simulink model "test_darko"  (R2021b)
settings: Solver=VariableStepAuto  StartTime=0.0  StopTime=100  RelTol=1e-3
values from neighbouring files (symbols this model uses):
  initial_state = [p_initial; v_initial; q_initial; omega_initial]    [systune_gain_scheduling.m]    (also in systune_variable_gain_scheduling_LPV.m)
  u_eq = [ua;ua;ub;ub]    [systune_gain_scheduling.m]    (also in systune_variable_gain_scheduling_LPV.m)
  w = [0;0;0]    [systune_gain_scheduling.m]    (also in systune_variable_gain_scheduling_LPV.m = [-i;0;0])
libraries: simulink_extras x5, aerolibanim x1, sharedtransform x1
settings Model: Creator=florian  LastModifiedBy=florian
settings SolverCC: AlgebraicLoopSolver=TrustRegion
settings DebuggingCC: SFMachineParentedDataDiag=warning

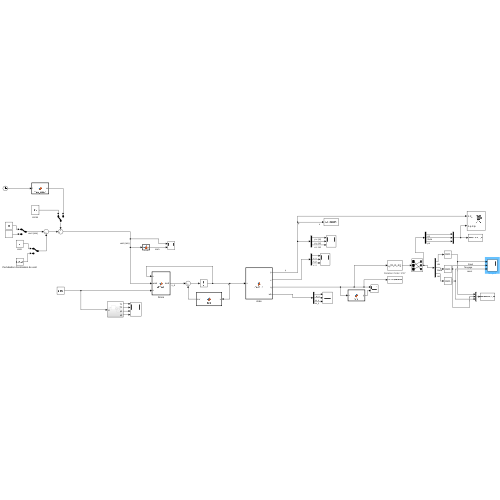
[thumbnail: Simulink's stored preview of the top-level diagram]
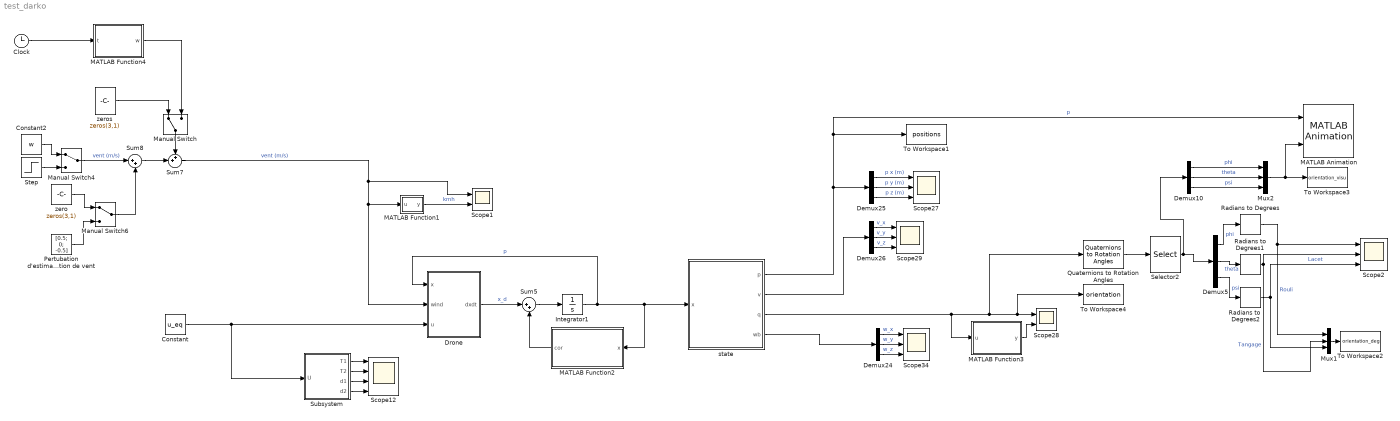
== system test_darko ==
  Clock : Clock
  Constant : Constant  Value=u_eq
  Constant2 : Constant  Value=w
  Demux{5,10,24..26} (5 alike) : Demux  Outputs=3
  Drone : MATLAB Function  TreatAsAtomicUnit=on
  Integrator1 : Integrator  InitialCondition=initial_state
  MATLAB Animation : aerolibanim/MATLAB Animation  Tag=Matlab Animation 6 DOF  Vehicles=1  Geometries='astredwedge.mat'  BoundingBoxCoordinates=[-50,50,-50,50,-50,50]  CameraOffset=[0,-50,0]  CameraViewAngle=10  SampleTime=0.08  FigurePosition=[635,-23,492,413]
      settings: SourceProductBaseCode=AE
  MATLAB Function1 : MATLAB Function  TreatAsAtomicUnit=on
  MATLAB Function2 : MATLAB Function  TreatAsAtomicUnit=on
  MATLAB Function3 : MATLAB Function  TreatAsAtomicUnit=on
  MATLAB Function4 : MATLAB Function  TreatAsAtomicUnit=on
  Manual Switch : ManualSwitch
  Manual Switch4 : ManualSwitch
  Manual Switch6 : ManualSwitch
  Mux1 : Mux  Inputs=3
  Mux2 : Mux  Inputs=3
  Pertubation d'estimation de vent : Constant  Value=[0.5; 0; -0.5]
  Quaternions to Rotation Angles : sharedtransform/Quaternions to Rotation Angles  rotationOrder=ZXY  aMode=aMode
      settings: SourceProductBaseCode=AE,PW,DR,MT,UV,VE
  Radians to Degrees : simulink_extras/Transformations/Radians to Degrees
  Radians to Degrees1 : simulink_extras/Transformations/Radians to Degrees
  Radians to Degrees2 : simulink_extras/Transformations/Radians to Degrees
  Scope1 : Scope  NumInputPorts=2
  Scope12 : Scope  NumInputPorts=4
  Scope{2,27,29,34} (4 alike) : Scope  NumInputPorts=3
  Scope28 : Scope  NumInputPorts=2
  Selector2 : Selector  InputPortWidth=3  IndexOptions=Index vector (dialog)  Indices=[2 3 1]  OutputSizes=1
  Step : Step  Time=20  Before=[0;0;0]  After=[-7;0;0]  SampleTime=0
  Subsystem : Subsystem
  Sum5 : Sum  Inputs=|++
  Sum7 : Sum  Inputs=++|
  Sum8 : Sum  Inputs=|++
  To Workspace1 : ToWorkspace  VariableName=positions  SampleTime=-1
  To Workspace2 : ToWorkspace  VariableName=orientation_deg  SampleTime=-1
  To Workspace3 : ToWorkspace  VariableName=orientation_visu  SampleTime=-1
  To Workspace4 : ToWorkspace  VariableName=orientation  SampleTime=-1
  state : MATLAB Function  TreatAsAtomicUnit=on
  zero : Constant  Value=zeros(3,1)
  zeros : Constant  Value=zeros(3,1)
  wires:
  Sum5/1 -> Integrator1/1
  MATLAB Function2/1(cor) -> Sum5/2
  Drone/1(dxdt) -> Sum5/1  "x_d"
  Demux25/3 -> Scope27/3  "p z (m)"
  Demux26/2 -> Scope29/2  "v_y"
  Demux24/1 -> Scope34/1  "w_x"
  MATLAB Function3/1(y) -> Scope28/2
  Demux25/1 -> Scope27/1  "p x (m)"
  state/4(wb) -> Demux24/1
  Demux24/2 -> Scope34/2  "w_y"
  Demux24/3 -> Scope34/3  "w_z"
  state/2(v) -> Demux26/1
  Demux25/2 -> Scope27/2  "p y (m)"
  Demux26/3 -> Scope29/3  "v_z"
  Demux26/1 -> Scope29/1  "v_x"
  Demux5/2 -> Radians to Degrees1/1  "theta"
  Demux5/1 -> Radians to Degrees/1  "phi"
  Demux5/3 -> Radians to Degrees2/1  "psi"
  Mux1/1 -> To Workspace2/1
  state/3(q) -> Quaternions to Rotation Angles/1, Scope28/1, To Workspace4/1, MATLAB Function3/1(u)
  Demux10/2 -> Mux2/2  "theta"
  Selector2/1 -> Demux10/1, Demux5/1
  Demux10/1 -> Mux2/1  "phi"
  Demux10/3 -> Mux2/3  "psi"
  state/1(p) -> Demux25/1, MATLAB Animation/1, To Workspace1/1  "p"
  Mux2/1 -> To Workspace3/1, MATLAB Animation/2
  Sum7/1 -> Drone/2(wind), MATLAB Function1/1(u), Scope1/1  "vent (m/s)"
  Radians to Degrees1/1 -> Mux1/2, Scope2/2  "Tangage"
  Radians to Degrees/1 -> Scope2/1, Mux1/1  "Rouli"
  Radians to Degrees2/1 -> Scope2/3, Mux1/3  "Lacet"
  Step/1 -> Manual Switch4/2
  Constant2/1 -> Manual Switch4/1
  MATLAB Function1/1(y) -> Scope1/2  "kmh"
  Quaternions to Rotation Angles/1 -> Selector2/1
  Clock/1 -> MATLAB Function4/1(t)
  Integrator1/1 -> Drone/1(x), state/1(x), MATLAB Function2/1(x)  "p"
  Subsystem/1(T1) -> Scope12/1
  Subsystem/3(d1) -> Scope12/3
  Constant/1 -> Subsystem/1(U), Drone/3(u)
  Subsystem/2(T2) -> Scope12/2
  Subsystem/4(d2) -> Scope12/4
  Manual Switch/1 -> Sum7/1
  MATLAB Function4/1(w) -> Manual Switch/2
  zeros/1 -> Manual Switch/1
  Sum8/1 -> Sum7/2
  Manual Switch4/1 -> Sum8/1  "vent (m/s)"
  Pertubation d'estimation de vent/1 -> Manual Switch6/2
  Manual Switch6/1 -> Sum8/2
  zero/1 -> Manual Switch6/1

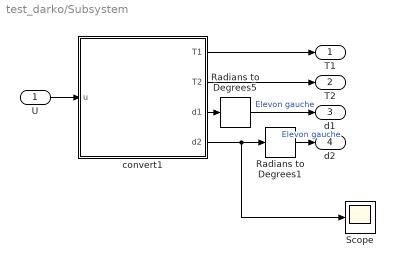
== system test_darko/Subsystem ==
  U : Inport
  Radians to Degrees1 : simulink_extras/Transformations/Radians to Degrees
  Radians to Degrees5 : simulink_extras/Transformations/Radians to Degrees
  Scope : Scope
  convert1 : MATLAB Function  TreatAsAtomicUnit=on
  T1 : Outport
  T2 : Outport  Port=2
  d1 : Outport  Port=3
  d2 : Outport  Port=4
  wires:
  U/1 -> convert1/1(u)
  convert1/1(T1) -> T1/1
  convert1/2(T2) -> T2/1
  Radians to Degrees5/1 -> d1/1  "Elevon gauche"
  convert1/3(d1) -> Radians to Degrees5/1
  Radians to Degrees1/1 -> d2/1  "Elevon gauche"
  convert1/4(d2) -> Scope/1, Radians to Degrees1/1

== matlab function test_darko/Drone ==
  data: x input; wind input; u input; dxdt output; drone parameter
function dxdt  = drone(x,wind, u, drone)

%% physical constants
% gravity
g = drone.G;
% vehicle mass
m = drone.MASS;
% vehicle inertia matrix
J = drone.INERTIA; % [3x3 real symmetric] in body axis

%% state demultiplexing
% p = x(1:3);
v = x(4:6);
q  = x(7:10);
wb = x(11:13);

Rq = q2dcm(q);

[Fp, Mp] = external_force_moment(x, u, wind, drone);

% position
dpdt = v;

% kinematics
dvdt =  [0;0;g] + (1/m)*Rq*drone.Fb*u + (1/m)*Rq*Fp; 

%% quaternion derivative
eta = q(1);
eps = q(2:4);

dqdt = (1/2)*[-eps'; eta*eye(3) + skew_sym(eps)]*wb;

%% angular velocity derivative
% kinematics
dwdt = -J\cross(wb, J*wb) + J\(drone.Mb*u) + J\Mp;


%% derivative multiplexing
dxdt = [dpdt; dvdt; dqdt; dwdt] ;

== matlab function test_darko/Subsystem/convert1 ==
  data: u input; T1 output; drone parameter; T2 output; d1 output; d2 output
function [T1, T2, d1, d2] = convert(u, drone)
%#codegen
kf = drone.PROP_KP;

T1 = max(u(1),0);
T2 = max(u(2),0);
d1_T1 = u(3);
d2_T2 = u(4);

w1 = sqrt(T1/kf);
w2 = sqrt(T2/kf);
d1 = d1_T1/T1;
d2 = d2_T2/T2;

== matlab function test_darko/MATLAB Function1 ==
  data: u input; y output
function y = nor(u)
%#codegen

y = norm(u)*3.6;

== matlab function test_darko/MATLAB Function4 ==
  data: t input; w output
function w = mex_wind(t)
%#codegen
t0 = 60; %s
wx_mean = 0;
fg = 0.8;
Ag = -1; %m/s
if (t-t0)<0 ||  (t-t0)> 1/fg
    wx = wx_mean;
else
    wx = wx_mean + (Ag/2)*(1-cos(2*pi*fg*(t-t0)))*sin(3*pi*fg*(t-t0));
end
w = [-wx;0;0];

== matlab function test_darko/MATLAB Function2 ==
  data: x input; cor output
function cor  = fcn(x)
%#codegen
q  = x(7:10);
n = norm(q);
mismatch = 1-n;
cor = [0;0;0; 0;0;0; mismatch*q; 0;0;0];

== matlab function test_darko/MATLAB Function3 ==
  data: u input; y output
function y = fcn(u)
%#codegen

y = norm(u);

== matlab function test_darko/state ==
  data: x input; p output; v output; q output; wb output
function [p, v, q, wb] = demux(x)
%#codegen

p = x(1:3);
v = x(4:6);
q  = x(7:10);
wb = x(11:13);
